simulink model "lab4_PID_2"  (R2019b)
settings: Solver=VariableStepAuto  StartTime=0.0  StopTime=10.0  RelTol=1e-3
values from neighbouring files (symbols this model uses):
  angle_1 = 3.14    [lab4.m]
  J = 0.0023    [lab4.m]
  Kb = 5    [lab4.m]
  Kd = 0.03    [lab4.m]
  Ke = Km    (= 0.29)    [lab4.m]
  Ki = 0.05    [lab4.m]
  Km = 0.29    [lab4.m]
  Kp = 3    [lab4.m]
  L = 0.0047    [lab4.m]
  R = 4.7    [lab4.m]
  Um = 3.5    [lab4.m]
libraries: simulink x1
settings Model: Creator=Ivan  LastModifiedBy=Ivan

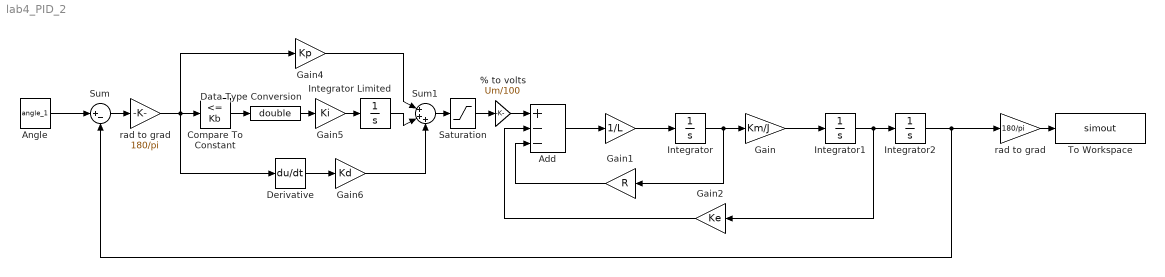
== system lab4_PID_2 ==
  " " : Gain  Gain=1/L
  % to volts : Gain  Gain=Um/100
  Add : Sum  Inputs=+--
  Angle : Constant  Value=angle_1  VectorParams1D=off
  Compare To Constant : simulink/Logic and Bit Operations/Compare To Constant  relop=<=  const=Kb  OutDataTypeStr=boolean
  Data Type Conversion : DataTypeConversion  OutMin=[0]  OutMax=[1]  OutDataTypeStr=double
  Derivative : Derivative
  Gain : Gain  Gain=Km/J
  Gain1 : Gain  Gain=R
  Gain2 : Gain  Gain=Ke
  Gain4 : Gain  Gain=Kp
  Gain5 : Gain  Gain=Ki
  Gain6 : Gain  Gain=Kd
  Integrator : Integrator
  Integrator Limited : Integrator  LimitOutput=on
  Integrator1 : Integrator
  Integrator2 : Integrator
  Saturation : Saturate  UpperLimit=100  LowerLimit=-100
  Sum : Sum  Inputs=|+-
  Sum1 : Sum  Inputs=|+++
  To Workspace : ToWorkspace  VariableName=simout  SaveFormat=Timeseries  SampleTime=-1
  rad to grad : Gain  Gain=180/pi
  "rad to grad " : Gain  Gain=180/pi
  wires:
  Integrator2/1 -> "rad to grad "/1, Sum/2
  "rad to grad "/1 -> To Workspace/1
  Gain2/1 -> Add/2
  % to volts/1 -> Add/1
  Gain/1 -> Integrator1/1
  Add/1 -> " "/1
  Gain1/1 -> Add/3
  " "/1 -> Integrator/1
  Integrator1/1 -> Gain2/1, Integrator2/1
  Integrator/1 -> Gain1/1, Gain/1
  Sum/1 -> rad to grad/1
  Angle/1 -> Sum/1
  Gain4/1 -> Sum1/1
  Derivative/1 -> Gain6/1
  Gain6/1 -> Sum1/3
  rad to grad/1 -> Compare To Constant/1, Derivative/1, Gain4/1
  Gain5/1 -> Integrator Limited/1
  Integrator Limited/1 -> Sum1/2
  Compare To Constant/1 -> Data Type Conversion/1
  Data Type Conversion/1 -> Gain5/1
  Sum1/1 -> Saturation/1
  Saturation/1 -> % to volts/1
